simulink model "thrusters_model"  (R2019b)
settings: Solver=FixedStepAuto  StartTime=0.0  StopTime=500  FixedStep=0.001  RelTol=1e-3
values from neighbouring files (symbols this model uses):
  a0 = 0.5    [rw_script.m]    (also in thrusters_script.m)
  a1 = 3    [rw_script.m]    (also in thrusters_script.m)
  I = 10    [rw_script.m]    (also in thrusters_script.m = 1)
  Kd = 0.1    [rw_script.m]    (also in thrusters_script.m = 2)
  Kp = 1    [rw_script.m]    (also in thrusters_script.m = 0.5)
  mag_sat = 1    [rw_script.m]    (also in thrusters_script.m = 0.005)
  thrust = 1    [rw_script.m]    (also in thrusters_script.m = 0.5)
libraries: simulink x1
settings Model: Creator=asmialek  LastModifiedBy=asmialek
settings DataIOCC: SaveOutput=off  SignalLogging=off  DSMLogging=off  ReturnWorkspaceOutputs=off

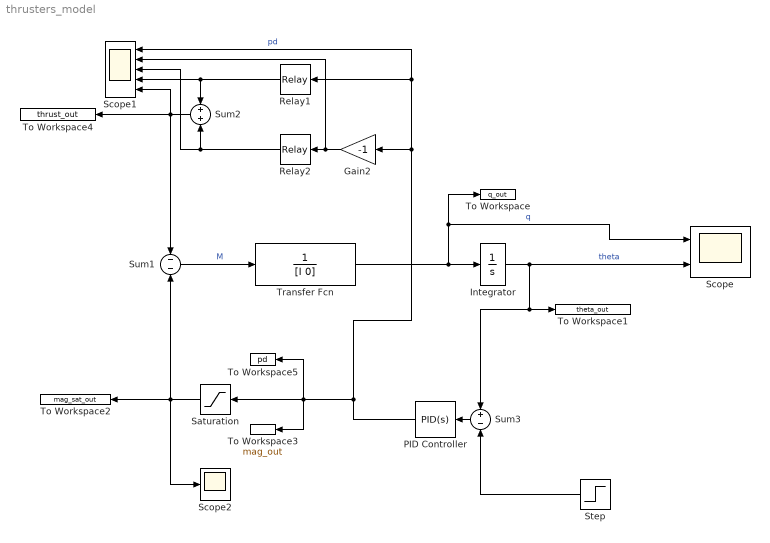
== system thrusters_model ==
  Gain2 : Gain  Gain=-1
  Integrator : Integrator
  PID Controller : simulink/Continuous/PID Controller  Controller=PID  Form=Parallel  TimeDomain=Continuous-time  SampleTime=-1  IntegratorMethod=Forward Euler  FilterMethod=Forward Euler  ControllerParametersSource=internal  P=Kp  I=0  D=Kd  UseFilter=on  N=100  TunerSelectOption=Transfer Function Based (PID Tuner App)  InitialConditionSource=internal  InitialConditionForIntegrator=0  InitialConditionForFilter=0  DifferentiatorICPrevScaledInput=0  ExternalReset=none  TrackingMode=off  Kt=1  LimitOutput=off  UpperSaturationLimit=inf  LowerSaturationLimit=-inf  LinearizeAsGain=on  AntiWindupMode=none  Kb=1  POutMin=[]  POutMax=[]  IOutMin=[]  IOutMax=[]  DOutMin=[]  DOutMax=[]  NOutMin=[]  NOutMax=[]  SumOutMin=[]  SumOutMax=[]  SaturationOutMin=[]  SaturationOutMax=[]  PParamMin=[]  PParamMax=[]  IParamMin=[]  IParamMax=[]  DParamMin=[]  DParamMax=[]  NParamMin=[]  NParamMax=[]  KbParamMin=[]  KbParamMax=[]  KtParamMin=[]  KtParamMax=[]  KbOutMin=[]  KbOutMax=[]  KtOutMin=[]  KtOutMax=[]  IntegratorOutMin=[]  IntegratorOutMax=[]  FilterOutMin=[]  FilterOutMax=[]  SumI1OutMin=[]  SumI1OutMax=[]  SumI2OutMin=[]  SumI2OutMax=[]  SumI3OutMin=[]  SumI3OutMax=[]  SumI4OutMin=[]  SumI4OutMax=[]  SumDOutMin=[]  SumDOutMax=[]  DifferentiatorOutMin=[]  DifferentiatorOutMax=[]  FilterDiffOutCoefMin=[]  FilterDiffOutCoefMax=[]  ReciprocalOutMin=[]  ReciprocalOutMax=[]  SumDenOutMin=[]  SumDenOutMax=[]  SumNumOutMin=[]  SumNumOutMax=[]  DivideOutMin=[]  DivideOutMax=[]  IntegratorContinuousStateAttributes=''  IntegratorStateMustResolveToSignalObject=off  IntegratorRTWStateStorageClass=Auto  FilterContinuousStateAttributes=''  FilterStateMustResolveToSignalObject=off  FilterRTWStateStorageClass=Auto  ParallelPVariant=InternalParameters  IdealPVariant=Disabled  IVariant=InternalParameters  DVariant=InternalParameters  IntegratorVariant=Continuous  SatVariant=Disabled  AWVariant=Passthrough  PCopyVariant=Disabled  TRVariant=Disabled  FdbkBlocksVariant=Forward  IdealPFdbkVariant=Disabled  SatFdbkVariant=Disabled  DerivativeFilterVariant=ContFilter  NVariant=InternalParameters  NCopyVariant=Disabled  FilterICVariant=InternalICsFilter  IntegratorICVariant=InternalICs  ExternalResetVariant=Disabled  TRSumVariant=Passthrough  SumFdbkVariant=Disabled  SumVariant=Sum_PID
  Relay1 : Relay  OnSwitchValue=a1  OffSwitchValue=a0  OnOutputValue=thrust
  Relay2 : Relay  OnSwitchValue=a1  OffSwitchValue=a0  OnOutputValue=-thrust
  Saturation : Saturate  UpperLimit=mag_sat  LowerLimit=-mag_sat
  Scope : Scope  NumInputPorts=2
  Scope1 : Scope  NumInputPorts=5
  Scope2 : Scope
  Step : Step  Time=20  After=20  SampleTime=0
  Sum1 : Sum  Inputs=-|-
  Sum2 : Sum  Inputs=+|+
  Sum3 : Sum  Inputs=+-
  To Workspace : ToWorkspace  VariableName=q_out  SampleTime=-1
  To Workspace1 : ToWorkspace  VariableName=theta_out  SampleTime=-1
  To Workspace2 : ToWorkspace  VariableName=mag_sat_out  SampleTime=-1
  To Workspace3 : ToWorkspace  VariableName=mag_out  SampleTime=-1
  To Workspace4 : ToWorkspace  VariableName=thrust_out  SampleTime=-1
  To Workspace5 : ToWorkspace  VariableName=pd  SampleTime=-1
  Transfer Fcn : TransferFcn  Denominator=[I 0]
  wires:
  PID Controller/1 -> Scope1/1, Relay1/1, Gain2/1, Saturation/1, To Workspace3/1, To Workspace5/1  "pd"
  Transfer Fcn/1 -> Scope/1, To Workspace/1, Integrator/1  "q"
  Integrator/1 -> To Workspace1/1, Sum3/1, Scope/2  "theta"
  Sum1/1 -> Transfer Fcn/1  "M"
  Saturation/1 -> Sum1/2, Scope2/1, To Workspace2/1
  Relay2/1 -> Scope1/3, Sum2/2
  Relay1/1 -> Scope1/4, Sum2/1
  Gain2/1 -> Scope1/2, Relay2/1
  Sum2/1 -> Scope1/5, Sum1/1, To Workspace4/1
  Step/1 -> Sum3/2
  Sum3/1 -> PID Controller/1
